simulink model "car_sim"  (R2013b)
settings: Solver=ode4  StartTime=0.0  StopTime=15  FixedStep=0.001  RelTol=1e-3
values from neighbouring files (symbols this model uses):
  n = 1834    [car.m]
  r = 0.078    [car.m]
  w = 0.393    [car.m]
libraries: simulink x4
settings Model: Creator=ShengChieh  LastModifiedBy=ShengChieh
settings DataIOCC: LimitDataPoints=off

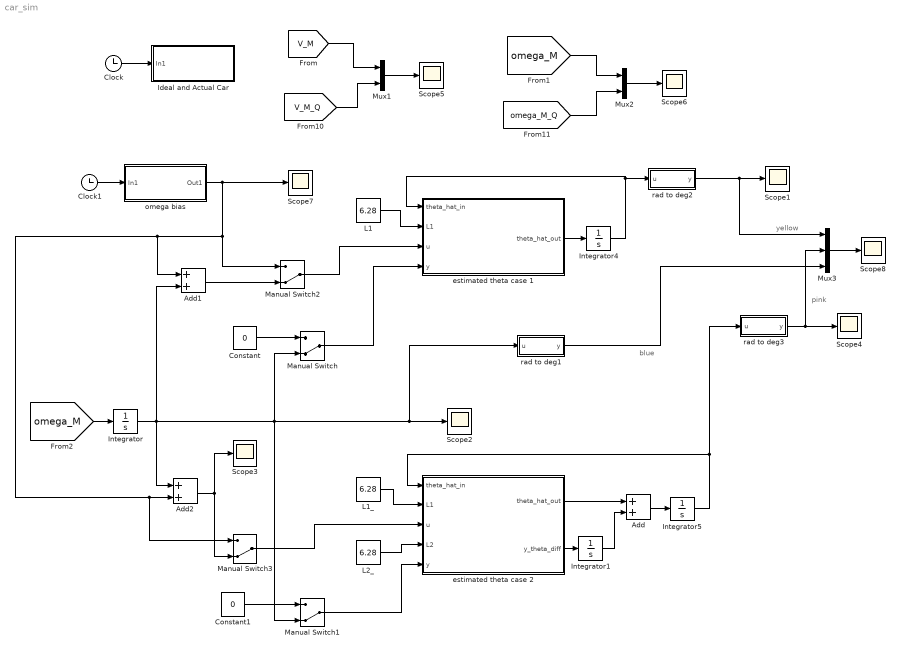
== system car_sim ==
  note: yellow
  note: pink
  note: blue
  Add : Sum
  Add1 : Sum
  Add2 : Sum
  Clock : Clock
  Clock1 : Clock
  Constant : Constant  Value=0
  Constant1 : Constant  Value=0
  Ideal and Actual Car : Subsystem
  Integrator{,1,4..5} (4 alike) : Integrator
  L1 : Constant  Value=6.28
  L1_ : Constant  Value=6.28
  L2_ : Constant  Value=6.28
  Manual Switch{,1..3} (4 alike) : ManualSwitch  CurrentSetting=0
  Mux1 : Mux  Inputs=2
  Mux2 : Mux  Inputs=2
  Mux3 : Mux  Inputs=3
  Scope{1..8} (8 alike) : Scope
      Scope1 settings: SaveName=ScopeData11
      Scope3 settings: SaveName=ScopeData3
      Scope4 settings: SaveName=ScopeData15
      Scope5 settings: SaveName=ScopeData16
      Scope6 settings: SaveName=ScopeData17
      Scope7 settings: SaveName=ScopeData18
      Scope8 settings: SaveName=ScopeData19
  estimated theta case 1 : MATLAB Function  TreatAsAtomicUnit=on
  estimated theta case 2 : MATLAB Function  TreatAsAtomicUnit=on
  omega bias : Subsystem  TreatAsAtomicUnit=on
  rad to deg1 : MATLAB Function  TreatAsAtomicUnit=on
  rad to deg2 : MATLAB Function  TreatAsAtomicUnit=on
  rad to deg3 : MATLAB Function  TreatAsAtomicUnit=on
  wires:
  Clock/1 -> Ideal and Actual Car/1(In1)
  estimated theta case 1/1(theta_hat_out) -> Integrator4/1
  Integrator4/1 -> estimated theta case 1/1(theta_hat_in), rad to deg2/1(u)
  L1/1 -> estimated theta case 1/2(L1)
  rad to deg2/1(y) -> Mux3/1, Scope1/1
  [V_M] -> Mux1/1
  [V_M_Q] -> Mux1/2
  Mux1/1 -> Scope5/1
  [omega_M] -> Mux2/1
  [omega_M_Q] -> Mux2/2
  Mux2/1 -> Scope6/1
  Clock1/1 -> omega bias/1(In1)
  estimated theta case 2/2(y_theta_diff) -> Integrator1/1
  Integrator1/1 -> Add/2
  estimated theta case 2/1(theta_hat_out) -> Add/1
  Add/1 -> Integrator5/1
  Integrator5/1 -> rad to deg3/1(u), estimated theta case 2/1(theta_hat_in)
  L1_/1 -> estimated theta case 2/2(L1)
  rad to deg3/1(y) -> Mux3/2, Scope4/1
  Mux3/1 -> Scope8/1
  L2_/1 -> estimated theta case 2/4(L2)
  Constant/1 -> Manual Switch/1
  Manual Switch/1 -> estimated theta case 1/4(y)
  Constant1/1 -> Manual Switch1/1
  Manual Switch1/1 -> estimated theta case 2/5(y)
  [omega_M] -> Integrator/1
  Integrator/1 -> Add2/1, Add1/2, Manual Switch1/2, Manual Switch/2, rad to deg1/1(u), Scope2/1
  rad to deg1/1(y) -> Mux3/3
  Manual Switch2/1 -> estimated theta case 1/3(u)
  Add1/1 -> Manual Switch2/2
  omega bias/1(Out1) -> Manual Switch2/1, Add1/1, Add2/2, Manual Switch3/1, Scope7/1
  Add2/1 -> Scope3/1, Manual Switch3/2
  Manual Switch3/1 -> estimated theta case 2/3(u)

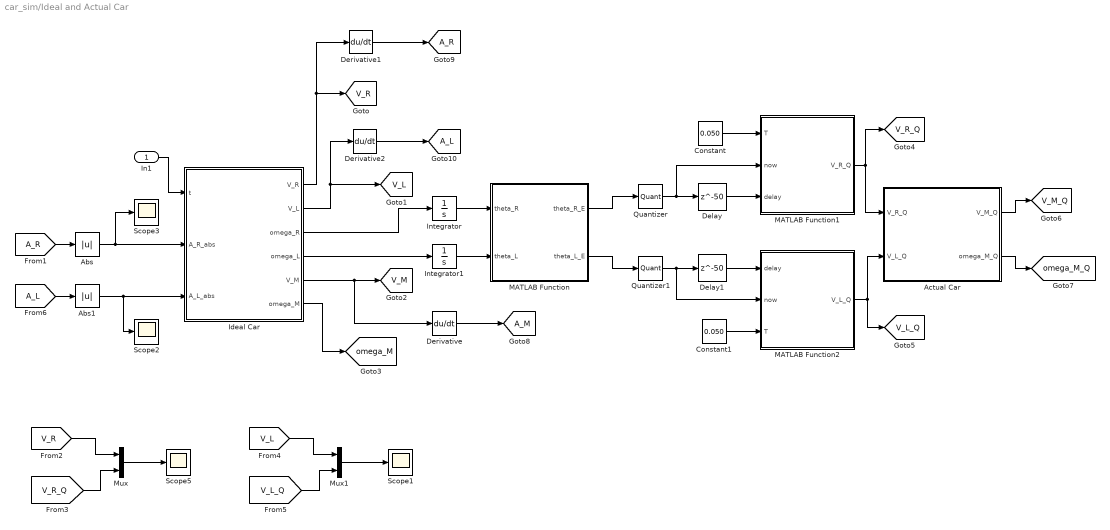
== system car_sim/Ideal and Actual Car ==
  In1 : Inport
  Abs : Abs
  Abs1 : Abs
  Actual Car : MATLAB Function  TreatAsAtomicUnit=on
  Constant : Constant  Value=0.050
  Constant1 : Constant  Value=0.050
  Delay : Delay  DelayLength=50
  Delay1 : Delay  DelayLength=50
  Derivative : Derivative
  Derivative1 : Derivative
  Derivative2 : Derivative
  Ideal Car : MATLAB Function  TreatAsAtomicUnit=on
  Integrator : Integrator
  Integrator1 : Integrator
  MATLAB Function : MATLAB Function  TreatAsAtomicUnit=on
  MATLAB Function1 : MATLAB Function  TreatAsAtomicUnit=on
  MATLAB Function2 : MATLAB Function  TreatAsAtomicUnit=on
  Mux : Mux  Inputs=2
  Mux1 : Mux  Inputs=2
  Quantizer : Quantizer  QuantizationInterval=1
  Quantizer1 : Quantizer  QuantizationInterval=1
  Scope{1..3,5} (4 alike) : Scope
      Scope1 settings: SaveName=ScopeData2
      Scope2 settings: SaveName=ScopeData12
      Scope3 settings: SaveName=ScopeData14
      Scope5 settings: TimeRange=10  YMin=-1  YMax=1
  tag scope: A_L=global, A_M=global, A_R=global, V_L=global, V_L_Q=global, V_M=global, V_M_Q=global, V_R=global, V_R_Q=global, omega_M=global, omega_M_Q=global
  wires:
  Ideal Car/1(V_R) -> Derivative1/1, [V_R]
  Ideal Car/2(V_L) -> Derivative2/1, [V_L]
  Ideal Car/3(omega_R) -> Integrator/1
  Ideal Car/4(omega_L) -> Integrator1/1
  Ideal Car/5(V_M) -> Derivative/1, [V_M]
  Ideal Car/6(omega_M) -> [omega_M]
  Integrator/1 -> MATLAB Function/1(theta_R)
  Integrator1/1 -> MATLAB Function/2(theta_L)
  Quantizer/1 -> MATLAB Function1/2(now), Delay/1
  Quantizer1/1 -> MATLAB Function2/2(now), Delay1/1
  Delay/1 -> MATLAB Function1/3(delay)
  Constant/1 -> MATLAB Function1/1(T)
  Delay1/1 -> MATLAB Function2/1(delay)
  Constant1/1 -> MATLAB Function2/3(T)
  MATLAB Function1/1(V_R_Q) -> Actual Car/1(V_R_Q), [V_R_Q]
  MATLAB Function2/1(V_L_Q) -> Actual Car/2(V_L_Q), [V_L_Q]
  Actual Car/1(V_M_Q) -> [V_M_Q]
  Actual Car/2(omega_M_Q) -> [omega_M_Q]
  Derivative/1 -> [A_M]
  In1/1 -> Ideal Car/1(t)
  [V_R] -> Mux/1
  [V_R_Q] -> Mux/2
  Mux/1 -> Scope5/1
  [V_L] -> Mux1/1
  [V_L_Q] -> Mux1/2
  Mux1/1 -> Scope1/1
  Derivative2/1 -> [A_L]
  Derivative1/1 -> [A_R]
  [A_R] -> Abs/1
  [A_L] -> Abs1/1
  Abs/1 -> Scope3/1, Ideal Car/2(A_R_abs)
  Abs1/1 -> Ideal Car/3(A_L_abs), Scope2/1
  MATLAB Function/1(theta_R_E) -> Quantizer/1
  MATLAB Function/2(theta_L_E) -> Quantizer1/1

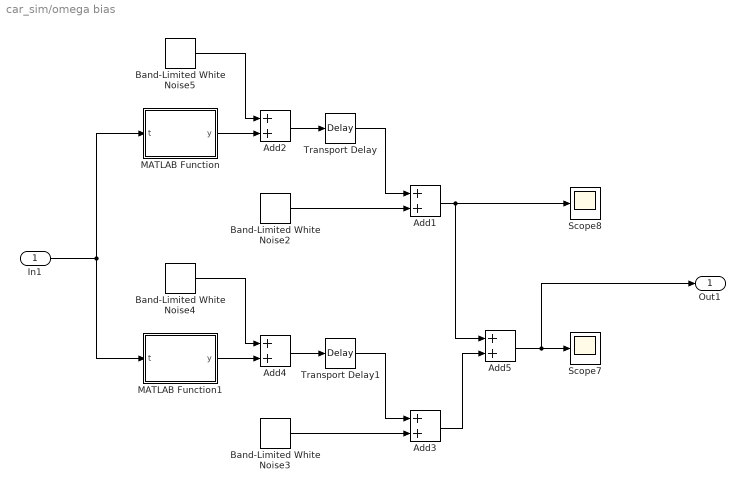
== system car_sim/omega bias ==
  In1 : Inport
  Add{1..5} (5 alike) : Sum
  Band-Limited White Noise{2..5} (4 alike) : simulink/Sources/Band-Limited White Noise  Cov=[0.00000001]  Ts=0.001  seed=[23341]
  MATLAB Function : MATLAB Function  TreatAsAtomicUnit=on
  MATLAB Function1 : MATLAB Function  TreatAsAtomicUnit=on
  Scope7 : Scope
      settings: SaveName=ScopeData7
  Scope8 : Scope
      settings: SaveName=ScopeData10
  Transport Delay : TransportDelay  DelayTime=4.5
  Transport Delay1 : TransportDelay  DelayTime=3.5
  Out1 : Outport
  wires:
  Band-Limited White Noise5/1 -> Add2/1
  MATLAB Function/1(y) -> Add2/2
  Add2/1 -> Transport Delay/1
  Transport Delay/1 -> Add1/1
  Band-Limited White Noise2/1 -> Add1/2
  Add1/1 -> Add5/1, Scope8/1
  Band-Limited White Noise4/1 -> Add4/1
  MATLAB Function1/1(y) -> Add4/2
  Add4/1 -> Transport Delay1/1
  Transport Delay1/1 -> Add3/1
  Band-Limited White Noise3/1 -> Add3/2
  Add3/1 -> Add5/2
  Add5/1 -> Out1/1, Scope7/1
  In1/1 -> MATLAB Function/1(t), MATLAB Function1/1(t)

== matlab function car_sim/Ideal and Actual Car/MATLAB Function ==
  data: theta_R input; theta_R_E output; theta_L input; n parameter; theta_L_E output
function [theta_R_E,theta_L_E] = fcn(theta_R,theta_L,n)

theta_R_E = theta_R * n/(2*pi);    % rad to pulse
theta_L_E = theta_L * n/(2*pi);

== matlab function car_sim/Ideal and Actual Car/Ideal Car ==
  data: t input; V_R output; r parameter; w parameter; V_L output; omega_R output; omega_L output; V_M output; omega_M output; A_R_abs input; A_L_abs input
function [V_R,V_L,omega_R,omega_L,V_M,omega_M] = fcn(t,r,w,A_R_abs,A_L_abs)

V_R = 0.08*t^2 - 0.25*t - 0.5*sin(2.5*(t-3));
V_L = 0.08*t^2 - 0.30*t - 0.5*cos(2.2*(t-3));

% V_R = 0;
% V_L = 0;

V_M = (V_R + V_L) / 2;
omega_M = (V_R - V_L) / w;

% 以輪子半徑變形來模擬打滑 輪子半徑變形 正比於 扭力 or 加速度
r_R = r - A_R_abs/1.5*0.01;    %　限制輪子半徑變形不超過1cm
r_L = r - A_L_abs/1.5*0.01;
omega_R = V_R / r_R;
omega_L = V_L / r_L;

== matlab function car_sim/Ideal and Actual Car/MATLAB Function1 ==
  data: T input; V_R_Q output; now input; delay input; r parameter; n parameter
function V_R_Q = fcn(T,now,delay,r,n)

V_R_Q = (now - delay)/T * (2*pi)/n * r;

== matlab function car_sim/Ideal and Actual Car/MATLAB Function2 ==
  data: delay input; now input; T input; V_L_Q output; r parameter; n parameter
function V_L_Q = fcn(delay,now,T,r,n)

V_L_Q = (now - delay)/T * (2*pi)/n * r;

== matlab function car_sim/Ideal and Actual Car/Actual Car ==
  data: V_R_Q input; V_M_Q output; V_L_Q input; w parameter; omega_M_Q output
function [V_M_Q,omega_M_Q] = fcn(V_R_Q,V_L_Q,w)

V_M_Q = (V_R_Q + V_L_Q) / 2;
omega_M_Q = (V_R_Q - V_L_Q) / w;

== matlab function car_sim/rad to deg1 ==
  data: u input; y output
function y = fcn(u)

y = u*57.3;

== matlab function car_sim/rad to deg2 ==
  data: u input; y output
function y = fcn(u)

y = u*57.3;

== matlab function car_sim/omega bias/MATLAB Function ==
  data: t input; y output
function y = fcn(t)

y = -0.035*(t) + 0.002*(t)^2 + 0.000001*(t)^3;

== matlab function car_sim/estimated theta case 1 ==
  data: theta_hat_in input; L1 input; u input; y input; theta_hat_out output
function theta_hat_out = fcn(theta_hat_in,L1,u,y)

theta_hat_out = u + L1*(y - theta_hat_in);

== matlab function car_sim/omega bias/MATLAB Function1 ==
  data: t input; y output
function y = fcn(t)

y = -0.035*(t) + 0.002*(t)^2 + 0.000001*(t)^3;

== matlab function car_sim/estimated theta case 2 ==
  data: theta_hat_in input; L1 input; u input; L2 input; y input; theta_hat_out output; y_theta_diff output
function [theta_hat_out , y_theta_diff] = fcn(theta_hat_in,L1,u,L2,y)

theta_hat_out = u + L1*(y - theta_hat_in);

y_theta_diff = L2*(y - theta_hat_in);

== matlab function car_sim/rad to deg3 ==
  data: u input; y output
function y = fcn(u)

y = u*57.3;
